simulink model "untitled1"  (R2021a)
settings: Solver=VariableStepAuto  StartTime=0.0  StopTime=10.0  RelTol=1e-3
undefined symbols (not defined in the file or in its folder): Rec, SDTV
libraries: visionconversions x3, visiontransforms x2, visionanalysis x1, visionsources x1
settings Model: Creator=amorales  LastModifiedBy=amorales

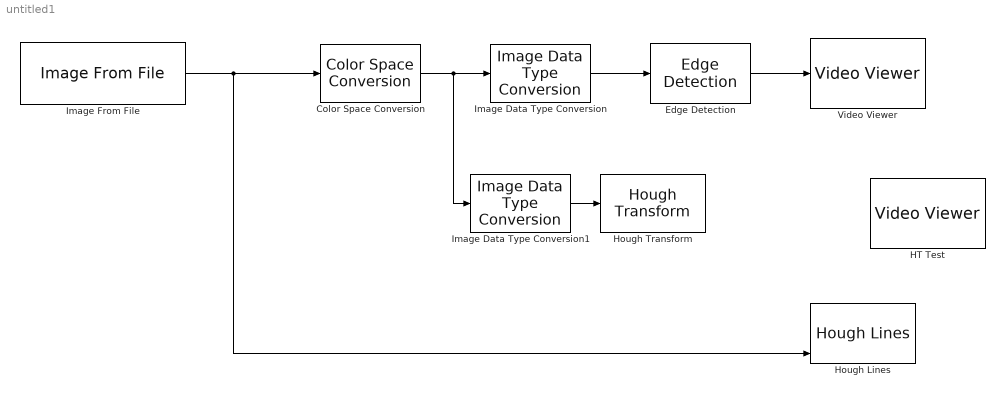
== system untitled1 ==
  Color Space Conversion : visionconversions/Color Space  Conversion  conversion=Obsolete  conversionActive=R'G'B' to intensity  wp_str=D65  rec=Rec. 601 (SDTV)  sys=1125/60/2:1  imagePorts=One multidimensional signal
  Edge Detection : visionanalysis/Edge Detection  method=Canny  outputType=Binary image  userDefinedThreshold=off  thresholdSource=Input port  threshold=20  thresholdTuning=4  edgeThinning=off  threshold_canny=[0.25 0.60]  autoPercent=70  sigma=1  roundingMode=Floor  overflowMode=off  prodOutputMode=Binary point scaling  prodOutputWordLength=32  prodOutputFracLength=8
      settings: SourceProductBaseCode=VP
  HT Test : VideoViewer  FigPos=[242 733 902 461]
  Hough Lines : visiontransforms/Hough Lines  sineCompMethod=Table lookup  thetaRes=pi/180  roundingMode=Nearest  overflowMode=on  firstCoeffMode=Specify word length  firstCoeffWordLength=16  prodOutputMode=Binary point scaling  prodOutputWordLength=32  prodOutputFracLength=16  firstCoeffFracLength=15
      settings: SourceProductBaseCode=VP
  Hough Transform : visiontransforms/Hough Transform  theta_res=pi/180  rho_res=1  out_theta_rho=off  outdtmode=double  roundingMode=Nearest  overflowMode=on  firstCoeffMode=Binary point scaling  firstCoeffWordLength=16  firstCoeffFracLength=14  secondCoeffMode=Binary point scaling  secondCoeffWordLength=32  secondCoeffFracLength=16  prodOutputMode=Binary point scaling  prodOutputWordLength=32  prodOutputFracLength=20  accumMode=Binary point scaling  accumWordLength=32  accumFracLength=20  outputMode=Binary point scaling  outputWordLength=16  outputFracLength=0  memoryMode=Binary point scaling  memoryWordLength=32  memoryFracLength=16
      settings: SourceProductBaseCode=VP
  Image Data Type Conversion : visionconversions/Image Data Type Conversion  outDT=single  isSigned=on  wordLen=16  numFracBits=0
      settings: SourceProductBaseCode=VP
  Image Data Type Conversion1 : visionconversions/Image Data Type Conversion  outDT=boolean  isSigned=on  wordLen=16  numFracBits=0
      settings: SourceProductBaseCode=VP
  Image From File : visionsources/Image From File  Tag=vipblks_nd  FileName=/Users/amorales/Documents/code/templates-robocup-robot-manipulation-challenge/MATLAB_Simulink_Templates/2021/Vision/data/1.jpeg  Ts=inf  imagePorts=One multidimensional signal  OutPortLabels=R|G|B  ImageDataType=Inherit from input image  sdImageDataType=uint(8)  Signed=on  WordLength=16  FractionLengthMode=User-defined  FractionLength=15
  Video Viewer : VideoViewer  FigPos=[461 898 974 564]
  wires:
  Edge Detection/1 -> Video Viewer/1
  Image From File/1 -> Color Space Conversion/1, Hough Lines/3
  Image Data Type Conversion/1 -> Edge Detection/1
  Color Space Conversion/1 -> Image Data Type Conversion1/1, Image Data Type Conversion/1
  Image Data Type Conversion1/1 -> Hough Transform/1
